simulink model "frt_dqpll"  (R2025b)
settings: Solver=ode23tb  StartTime=0.0  StopTime=simlength  FixedStep=tc  MaxStep=tc
values from neighbouring files (symbols this model uses):
  Adrso = eye(2) + Arso*ts_afe    [init_model.m]
  afe_pwm_phase_shift_mod1 = 0    [init_model.m]
  Crso = [1 0]    [init_model.m]
  delta_fht1 = 0.05    [init_model.m]
  frt_data = frt_settings(test_index, test_subindex, asymmetric_error_type, enable_frt_1, enable_frt_2, start_time_LVRT)    [init_model.m]
  grid_emu_data = grid_emulator(nominal_power, application_voltage, vp_xi_pu, vn_xi_pu, vn_eta_pu)    [init_model.m]
  i_grid_neg_eta_lim = 0.5    [init_model.m]
  i_grid_neg_eta_red_lim = 0.1    [init_model.m]
  i_grid_neg_xi_lim = 0.5    [init_model.m]
  i_grid_neg_xi_red_lim = 0.1    [init_model.m]
  i_grid_pos_eta_lim = 1    [init_model.m]
  i_grid_pos_eta_red_lim = 0.1    [init_model.m]
  ieta_neg_ref_lim = 0.5    [init_model.m]
  ieta_pos_ref_lim = 1.0    (= 1)    [init_model.m]
  ki_rc_neg_grid = ki_rc_grid    (= 35)    [init_model.m]
  ki_rc_pos_grid = ki_rc_grid    (= 35)    [init_model.m]
  kp_rc_neg_grid = kp_rc_grid    (= 0.35)    [init_model.m]
  kp_rc_pos_grid = kp_rc_grid    (= 0.35)    [init_model.m]
  Ld_fht1 = acker(Ad_fht1',Cfht1', polesd_fht1)    [init_model.m]
  Ldrso = acker(Adrso',Crso',polesdrso)'    [init_model.m]
  mavarage_filter_frequency_base_order = 2    [init_model.m]
  n1 = 2*pi*rms_perios/grid_emu_data.w_grid/ts_afe    [init_model.m]
  n10 = 2*pi*rms_perios/grid_emu_data.w_grid/ts_afe    [init_model.m]
  omega_f = grid_emu_data.w_grid    [init_model.m]
  omega_fht1 = grid_emu_data.w_grid    [init_model.m]
  pll_i1 = 80    [init_model.m]
  pll_i1_ddsrt = pll_i1    (= 80)    [init_model.m]
  pll_i1_fht = pll_i1    (= 80)    [init_model.m]
  pll_p = 1    [init_model.m]
  pll_p_ddsrt = pll_p    (= 1)    [init_model.m]
  pll_p_fht = pll_p    (= 1)    [init_model.m]
  pll_p_frt = 0.2    [init_model.m]
  start_time_LVRT = 0.75    [init_model.m]
  tc = ts_afe/400    (= 3.125e-07)    [init_model.m]
  time_gain_afe_module_1 = 1.0    (= 1)    [init_model.m]
  time_gain_inv_module_2 = 1.0    (= 1)    [init_model.m]
  ts_afe = 1/fPWM_AFE/2    (= 0.000125)    [init_model.m]
  vn_eta_pu = 0    [init_model.m]
  vn_xi_pu = 0    [init_model.m]
  vp_xi_pu = 1    [init_model.m]
  w_grid = grid_emu_data.w_grid    [init_model.m]
undefined symbols (not defined in the file or in its folder): g0_161Hz, g1_161Hz, LVRT_flt_ss_c, magnitude
libraries: fl_lib x42, nesl_utility x28, moving_average_filter x10, moving_average_filter_cc x8, cstblocks x7, discrete_time_low_pass_filter x4, simulink x3, single_phase_transformer_lib x3, linear_double_integrator_observer_ccaller x2, threephase_inductor_lib x1, power_meter_iec x1, three_phase_pwm_modulator x1
(part 4 of 6)

== system frt_dqpll/AFE_control/afe_control/grid_voltage_phase_lock_loops/dq_pll_ccaller/first_harmonic_tracker_phase_u ==
  u : Inport
  Bus Selector : BusSelector  OutputSignals=output_pu_hat
  C Caller : CCaller  FunctionName=first_harmonic_tracker_process_simulink  PortSpecificationStruct="%)30     .    B \\   8    (     @         %    \"     D    !     0         %  0 \"0    $    _    07)G3F%M90  4&]R=$YA;64 4V-O<&4     26YD97@     5'EP90      4VEZ90      27-';&]B86P   X    P    !@    @    $          4    (     0    ,    !         !   P!O=70 #@   #     &    \"     0         !0    @    !     P    $         $  # &]U=  .    .     8    (    !          %    \"     $    &     0         0  ...(+4988 chars)"
  Constant : Constant  Value=ts_afe
  Constant1 : Constant  Value=0
  Constant4 : Constant  Value=omega_fht1
  Constant5 : Constant  Value=delta_fht1
  Constant6 : Constant  Value=Ld_fht1(1)
  Constant7 : Constant  Value=Ld_fht1(2)
  Data Type Conversion{1..2,6..9} (6 alike) : DataTypeConversion  OutDataTypeStr=single  SaturateOnIntegerOverflow=off  RndMeth=Floor
  Data Type Conversion3 : DataTypeConversion  OutDataTypeStr=uint8  SaturateOnIntegerOverflow=off  RndMeth=Floor
  Data Type Conversion4 : DataTypeConversion  OutDataTypeStr=double  SaturateOnIntegerOverflow=off  RndMeth=Floor
  Data Type Conversion5 : DataTypeConversion  OutDataTypeStr=uint8  SaturateOnIntegerOverflow=off  RndMeth=Floor
  Step : Step  Time=0.0125  Before=1  After=0
  u_hat : Outport
  wires:
  Data Type Conversion4/1 -> u_hat/1
  Data Type Conversion3/1 -> C Caller/1
  Data Type Conversion1/1 -> C Caller/3
  Data Type Conversion2/1 -> C Caller/2
  C Caller/1 -> Bus Selector/1
  Bus Selector/1 -> Data Type Conversion4/1  "<output_pu_hat>"
  Step/1 -> Data Type Conversion3/1
  u/1 -> Data Type Conversion2/1
  Constant/1 -> Data Type Conversion1/1
  Constant1/1 -> Data Type Conversion5/1
  Constant4/1 -> Data Type Conversion6/1
  Constant6/1 -> Data Type Conversion8/1
  Constant7/1 -> Data Type Conversion9/1
  Constant5/1 -> Data Type Conversion7/1
  Data Type Conversion5/1 -> C Caller/8
  Data Type Conversion6/1 -> C Caller/4
  Data Type Conversion7/1 -> C Caller/5
  Data Type Conversion8/1 -> C Caller/6
  Data Type Conversion9/1 -> C Caller/7

== system frt_dqpll/AFE_control/afe_control/grid_voltage_phase_lock_loops/dq_pll_ccaller/first_harmonic_tracker_phase_v ==
  u : Inport
  Bus Selector : BusSelector  OutputSignals=output_pu_hat
  C Caller : CCaller  FunctionName=first_harmonic_tracker_process_simulink  PortSpecificationStruct="%)30     .    B \\   8    (     @         %    \"     D    !     0         %  0 \"0    $    _    07)G3F%M90  4&]R=$YA;64 4V-O<&4     26YD97@     5'EP90      4VEZ90      27-';&]B86P   X    P    !@    @    $          4    (     0    ,    !         !   P!O=70 #@   #     &    \"     0         !0    @    !     P    $         $  # &]U=  .    .     8    (    !          %    \"     $    &     0         0  ...(+4988 chars)"
  Constant : Constant  Value=ts_afe
  Constant1 : Constant  Value=2
  Constant4 : Constant  Value=omega_fht1
  Constant5 : Constant  Value=delta_fht1
  Constant6 : Constant  Value=Ld_fht1(1)
  Constant7 : Constant  Value=Ld_fht1(2)
  Data Type Conversion{1..2,6..9} (6 alike) : DataTypeConversion  OutDataTypeStr=single  SaturateOnIntegerOverflow=off  RndMeth=Floor
  Data Type Conversion3 : DataTypeConversion  OutDataTypeStr=uint8  SaturateOnIntegerOverflow=off  RndMeth=Floor
  Data Type Conversion4 : DataTypeConversion  OutDataTypeStr=double  SaturateOnIntegerOverflow=off  RndMeth=Floor
  Data Type Conversion5 : DataTypeConversion  OutDataTypeStr=uint8  SaturateOnIntegerOverflow=off  RndMeth=Floor
  Step : Step  Time=0.0125  Before=1  After=0
  u_hat : Outport
  wires:
  Data Type Conversion9/1 -> C Caller/7
  Data Type Conversion8/1 -> C Caller/6
  Data Type Conversion7/1 -> C Caller/5
  Data Type Conversion6/1 -> C Caller/4
  Data Type Conversion5/1 -> C Caller/8
  Constant5/1 -> Data Type Conversion7/1
  Constant7/1 -> Data Type Conversion9/1
  Constant6/1 -> Data Type Conversion8/1
  Constant4/1 -> Data Type Conversion6/1
  Constant1/1 -> Data Type Conversion5/1
  Constant/1 -> Data Type Conversion1/1
  u/1 -> Data Type Conversion2/1
  Step/1 -> Data Type Conversion3/1
  Bus Selector/1 -> Data Type Conversion4/1  "<output_pu_hat>"
  C Caller/1 -> Bus Selector/1
  Data Type Conversion2/1 -> C Caller/2
  Data Type Conversion1/1 -> C Caller/3
  Data Type Conversion3/1 -> C Caller/1
  Data Type Conversion4/1 -> u_hat/1

== system frt_dqpll/AFE_control/afe_control/grid_voltage_phase_lock_loops/dq_pll_ccaller/first_harmonic_tracker_phase_w ==
  u : Inport
  Bus Selector : BusSelector  OutputSignals=output_pu_hat
  C Caller : CCaller  FunctionName=first_harmonic_tracker_process_simulink  PortSpecificationStruct="%)30     .    B \\   8    (     @         %    \"     D    !     0         %  0 \"0    $    _    07)G3F%M90  4&]R=$YA;64 4V-O<&4     26YD97@     5'EP90      4VEZ90      27-';&]B86P   X    P    !@    @    $          4    (     0    ,    !         !   P!O=70 #@   #     &    \"     0         !0    @    !     P    $         $  # &]U=  .    .     8    (    !          %    \"     $    &     0         0  ...(+4988 chars)"
  Constant : Constant  Value=ts_afe
  Constant1 : Constant  Value=4
  Constant4 : Constant  Value=omega_fht1
  Constant5 : Constant  Value=delta_fht1
  Constant6 : Constant  Value=Ld_fht1(1)
  Constant7 : Constant  Value=Ld_fht1(2)
  Data Type Conversion{1..2,6..9} (6 alike) : DataTypeConversion  OutDataTypeStr=single  SaturateOnIntegerOverflow=off  RndMeth=Floor
  Data Type Conversion3 : DataTypeConversion  OutDataTypeStr=uint8  SaturateOnIntegerOverflow=off  RndMeth=Floor
  Data Type Conversion4 : DataTypeConversion  OutDataTypeStr=double  SaturateOnIntegerOverflow=off  RndMeth=Floor
  Data Type Conversion5 : DataTypeConversion  OutDataTypeStr=uint8  SaturateOnIntegerOverflow=off  RndMeth=Floor
  Step : Step  Time=0.0125  Before=1  After=0
  u_hat : Outport
  wires:
  Data Type Conversion4/1 -> u_hat/1
  Data Type Conversion3/1 -> C Caller/1
  Data Type Conversion1/1 -> C Caller/3
  Data Type Conversion2/1 -> C Caller/2
  C Caller/1 -> Bus Selector/1
  Bus Selector/1 -> Data Type Conversion4/1  "<output_pu_hat>"
  Step/1 -> Data Type Conversion3/1
  u/1 -> Data Type Conversion2/1
  Constant/1 -> Data Type Conversion1/1
  Constant1/1 -> Data Type Conversion5/1
  Constant4/1 -> Data Type Conversion6/1
  Constant6/1 -> Data Type Conversion8/1
  Constant7/1 -> Data Type Conversion9/1
  Constant5/1 -> Data Type Conversion7/1
  Data Type Conversion5/1 -> C Caller/8
  Data Type Conversion6/1 -> C Caller/4
  Data Type Conversion7/1 -> C Caller/5
  Data Type Conversion8/1 -> C Caller/6
  Data Type Conversion9/1 -> C Caller/7

== system frt_dqpll/AFE_control/afe_control/grid_voltage_sequences/voltage_sequence_avg/average_filter ==
  v_grid_pos_xi : Inport
  v_grid_pos_eta : Inport  Port=2
  v_grid_neg_xi : Inport  Port=3
  v_grid_neg_eta : Inport  Port=4
  Abs : Abs  SaturateOnIntegerOverflow=off
  Gain : Gain  Gain=grid_emu_data.omega_grid_nom*mavarage_filter_frequency_base_order
  Saturation : Saturate  UpperLimit=2  LowerLimit=0.1
  dmavg_flt{,1..3} (4 alike) : moving_average_filter/dmavg_flt  ts=ts_afe  enable_time=dmavg_filter_enable_time
  v_grid_pos_xi_avg : Outport
  v_grid_pos_eta_avg : Outport  Port=2
  v_grid_neg_xi_avg : Outport  Port=3
  v_grid_neg_eta_avg : Outport  Port=4
  wires:
  v_grid_neg_eta/1 -> dmavg_flt3/1
  v_grid_neg_xi/1 -> dmavg_flt2/1
  v_grid_pos_eta/1 -> dmavg_flt1/1
  dmavg_flt3/1 -> v_grid_neg_eta_avg/1
  dmavg_flt2/1 -> v_grid_neg_xi_avg/1
  dmavg_flt1/1 -> v_grid_pos_eta_avg/1
  Gain/1 -> dmavg_flt/2, dmavg_flt1/2, dmavg_flt2/2, dmavg_flt3/2
  dmavg_flt/1 -> v_grid_pos_xi_avg/1
  v_grid_pos_xi/1 -> dmavg_flt/1
  Abs/1 -> Saturation/1
  [omega_grid_pll_pu_mod1] -> Abs/1
  Saturation/1 -> Gain/1

== system frt_dqpll/AFE_control/afe_control/grid_voltage_sequences/voltage_sequence_avg/average_filter_ccaller ==
  v_grid_pos_xi : Inport
  v_grid_pos_eta : Inport  Port=2
  v_grid_neg_xi : Inport  Port=3
  v_grid_neg_eta : Inport  Port=4
  Abs : Abs  SaturateOnIntegerOverflow=off
  Gain : Gain  Gain=grid_emu_data.omega_grid_nom*mavarage_filter_frequency_base_order
  Saturation : Saturate  UpperLimit=2  LowerLimit=0.1
  dmavg_flt : moving_average_filter_cc/dmavg_flt  instance=0  ts=ts_afe  enable_time=dmavg_filter_enable_time
  dmavg_flt1 : moving_average_filter_cc/dmavg_flt  instance=1  ts=ts_afe  enable_time=dmavg_filter_enable_time
  dmavg_flt2 : moving_average_filter_cc/dmavg_flt  instance=2  ts=ts_afe  enable_time=dmavg_filter_enable_time
  dmavg_flt3 : moving_average_filter_cc/dmavg_flt  instance=3  ts=ts_afe  enable_time=dmavg_filter_enable_time
  v_grid_pos_xi_avg : Outport
  v_grid_pos_eta_avg : Outport  Port=2
  v_grid_neg_xi_avg : Outport  Port=3
  v_grid_neg_eta_avg : Outport  Port=4
  wires:
  v_grid_pos_xi/1 -> dmavg_flt/1
  dmavg_flt/1 -> v_grid_pos_xi_avg/1
  dmavg_flt1/1 -> v_grid_pos_eta_avg/1
  dmavg_flt2/1 -> v_grid_neg_xi_avg/1
  dmavg_flt3/1 -> v_grid_neg_eta_avg/1
  v_grid_pos_eta/1 -> dmavg_flt1/1
  v_grid_neg_xi/1 -> dmavg_flt2/1
  v_grid_neg_eta/1 -> dmavg_flt3/1
  Abs/1 -> Saturation/1
  Saturation/1 -> Gain/1
  [omega_grid_pll_pu_mod1] -> Abs/1
  Gain/1 -> dmavg_flt/2, dmavg_flt1/2, dmavg_flt3/2, dmavg_flt2/2

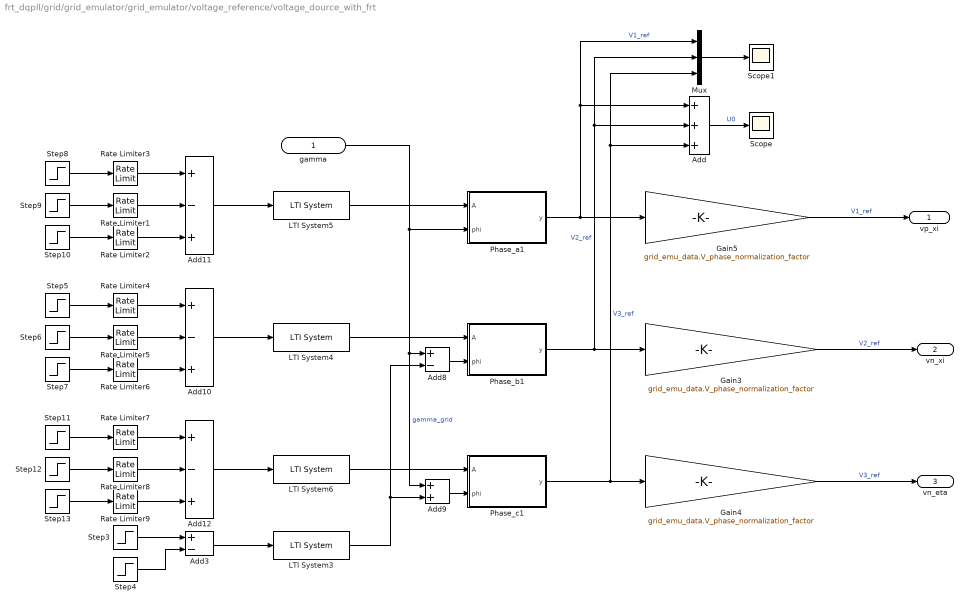
== system frt_dqpll/grid/grid_emulator/grid_emulator/voltage_reference/voltage_dource_with_frt ==
  gamma : Inport
  Add : Sum  Inputs=+++
  Add10 : Sum  Inputs=+-+
  Add11 : Sum  Inputs=+-+
  Add12 : Sum  Inputs=+-+
  Add3 : Sum  Inputs=+-
  Add8 : Sum  Inputs=+-
  Add9 : Sum
  Gain3 : Gain  Gain=grid_emu_data.V_phase_normalization_factor
  Gain4 : Gain  Gain=grid_emu_data.V_phase_normalization_factor
  Gain5 : Gain  Gain=grid_emu_data.V_phase_normalization_factor
  LTI System{3..6} (4 alike) : cstblocks/LTI System  sys=LVRT_flt_ss_c  IC=[0]  PadeOrder=0
  Mux : Mux  Inputs=3
  Phase_a1 : MATLAB Function  TreatAsAtomicUnit=on
  Phase_b1 : MATLAB Function  TreatAsAtomicUnit=on
  Phase_c1 : MATLAB Function  TreatAsAtomicUnit=on
  Rate Limiter{1..9} (9 alike) : RateLimiter  RisingSlewLimit=grid_emu_data.Vemu_ref_norm/frt_data.t_ramp  FallingSlewLimit=-grid_emu_data.Vemu_ref_norm/frt_data.t_ramp  SampleTimeMode=inherited
  Scope : Scope
      settings: ActiveDisplayYMinimum=-1E-15  ActiveDisplayYMaximum=8E-16
  Scope1 : Scope
      settings: ActiveDisplayYMinimum=-1.25511  ActiveDisplayYMaximum=1.25511
  Step10 : Step  Time=frt_data.end_time_LVRT  After=grid_emu_data.Vemu_ref_norm*(1-frt_data.Amplitude_U)  SampleTime=0
  Step11 : Step  Time=0  After=grid_emu_data.Vemu_ref_norm  SampleTime=0
  Step12 : Step  Time=frt_data.start_time_LVRT  After=grid_emu_data.Vemu_ref_norm*(1-frt_data.Amplitude_W)  SampleTime=0
  Step13 : Step  Time=frt_data.end_time_LVRT  After=grid_emu_data.Vemu_ref_norm*(1-frt_data.Amplitude_W)  SampleTime=0
  Step3 : Step  Time=frt_data.start_time_LVRT  After=frt_data.Phase_shift  SampleTime=0
  Step4 : Step  Time=frt_data.end_time_LVRT  After=frt_data.Phase_shift  SampleTime=0
  Step5 : Step  Time=0  After=grid_emu_data.Vemu_ref_norm  SampleTime=0
  Step6 : Step  Time=frt_data.start_time_LVRT  After=grid_emu_data.Vemu_ref_norm*(1-frt_data.Amplitude_V)  SampleTime=0
  Step7 : Step  Time=frt_data.end_time_LVRT  After=grid_emu_data.Vemu_ref_norm*(1-frt_data.Amplitude_V)  SampleTime=0
  Step8 : Step  Time=0  After=grid_emu_data.Vemu_ref_norm  SampleTime=0
  Step9 : Step  Time=frt_data.start_time_LVRT  After=grid_emu_data.Vemu_ref_norm*(1-frt_data.Amplitude_U)  SampleTime=0
  vp_xi : Outport  VectorParamsAs1DForOutWhenUnconnected=off
  vn_xi : Outport  Port=2  VectorParamsAs1DForOutWhenUnconnected=off
  vn_eta : Outport  Port=3  VectorParamsAs1DForOutWhenUnconnected=off
  wires:
  Phase_c1/1(y) -> Mux/3, Add/3, Gain4/1  "V3_ref"
  LTI System6/1 -> Phase_c1/1(A)
  gamma/1 -> Add9/1, Add8/1, Phase_a1/2(phi)  "gamma_grid"
  Add9/1 -> Phase_c1/2(phi)
  Add8/1 -> Phase_b1/2(phi)
  Phase_b1/1(y) -> Mux/2, Add/2, Gain3/1  "V2_ref"
  Phase_a1/1(y) -> Mux/1, Add/1, Gain5/1  "V1_ref"
  LTI System4/1 -> Phase_b1/1(A)
  Step5/1 -> Rate Limiter4/1
  Step6/1 -> Rate Limiter5/1
  Step7/1 -> Rate Limiter6/1
  Add10/1 -> LTI System4/1
  Step8/1 -> Rate Limiter3/1
  Add11/1 -> LTI System5/1
  Step9/1 -> Rate Limiter1/1
  Step10/1 -> Rate Limiter2/1
  LTI System5/1 -> Phase_a1/1(A)
  Add12/1 -> LTI System6/1
  Rate Limiter3/1 -> Add11/1
  Rate Limiter1/1 -> Add11/2
  Rate Limiter2/1 -> Add11/3
  Rate Limiter4/1 -> Add10/1
  Rate Limiter5/1 -> Add10/2
  Rate Limiter6/1 -> Add10/3
  Step12/1 -> Rate Limiter8/1
  Rate Limiter8/1 -> Add12/2
  Step13/1 -> Rate Limiter9/1
  Rate Limiter9/1 -> Add12/3
  Step11/1 -> Rate Limiter7/1
  Rate Limiter7/1 -> Add12/1
  Gain5/1 -> vp_xi/1  "V1_ref"
  Gain3/1 -> vn_xi/1  "V2_ref"
  Gain4/1 -> vn_eta/1  "V3_ref"
  Add3/1 -> LTI System3/1
  Step3/1 -> Add3/1
  Step4/1 -> Add3/2
  LTI System3/1 -> Add9/2, Add8/2
  Add/1 -> Scope/1  "U0"
  Mux/1 -> Scope1/1

== system frt_dqpll/grid/grid_emulator/three_phase_voltage_source_with_frt_emulator/three_phase_voltage_source_emulator/phase_gen1 ==
  Constant4 : Constant  Value=nominal_frequency_m*2*pi
  Integrator : Integrator
  bounder : MATLAB Function  TreatAsAtomicUnit=on  SystemSampleTime=ts_afe
  grid_emu_phase : Outport  VectorParamsAs1DForOutWhenUnconnected=off
  tag scope: gamma_grid_emulator=scoped, omega_grid_emulator=scoped
  wires:
  Integrator/1 -> bounder/1(u)
  Constant4/1 -> Integrator/1, [omega_grid_emulator]
  bounder/1(y) -> grid_emu_phase/1, [gamma_grid_emulator]  "grid_emu_phase"

== system frt_dqpll/grid/grid_emulator/three_phase_voltage_source_with_frt_emulator/three_phase_voltage_source_emulator/voltage_reference1 ==
  grid_emu_phase : Inport
  Vxi_p : Inport  Port=2
  Vxi_n : Inport  Port=3
  Veta_n : Inport  Port=4
  Constant2 : Constant  Value=0
  Sum1 : Sum  Inputs=|++
  Sum4 : Sum  Inputs=|++
  Variant Source : VariantSource  VariantControls={enable_frt_2_m == 1, enable_frt_1_m == 1}
  Variant Source1 : VariantSource  VariantControls={enable_frt_2_m == 1, enable_frt_1_m == 1}
  Variant Source2 : VariantSource  VariantControls={enable_frt_2_m == 1, enable_frt_1_m == 1}
  alphabeta2abc : MATLAB Function  TreatAsAtomicUnit=on  SystemSampleTime=ts_afe
  voltage_dource_with_frt : Subsystem
  xieta2alphabeta_neg : MATLAB Function  TreatAsAtomicUnit=on  SystemSampleTime=ts_afe
  xieta2alphabeta_pos : MATLAB Function  TreatAsAtomicUnit=on  SystemSampleTime=ts_afe
  V1_ref : Outport  VectorParamsAs1DForOutWhenUnconnected=off
  V2_ref : Outport  Port=2  VectorParamsAs1DForOutWhenUnconnected=off
  V3_ref : Outport  Port=3  VectorParamsAs1DForOutWhenUnconnected=off
  wires:
  [V3_ref_xieta] -> Variant Source2/1
  [V3_ref_abc] -> Variant Source2/2
  Variant Source2/1 -> V3_ref/1
  [V2_ref_abc] -> Variant Source1/2
  [V2_ref_xieta] -> Variant Source1/1
  Variant Source1/1 -> V2_ref/1
  [V1_ref_abc] -> Variant Source/2
  [V1_ref_xieta] -> Variant Source/1
  voltage_dource_with_frt/1(vp_xi) -> [V1_ref_abc]
  voltage_dource_with_frt/2(vn_xi) -> [V2_ref_abc]
  voltage_dource_with_frt/3(vn_eta) -> [V3_ref_abc]
  alphabeta2abc/3(c) -> [V3_ref_xieta]
  alphabeta2abc/2(b) -> [V2_ref_xieta]
  alphabeta2abc/1(a) -> [V1_ref_xieta]
  Variant Source/1 -> V1_ref/1
  Veta_n/1 -> xieta2alphabeta_neg/2(eta)
  Vxi_n/1 -> xieta2alphabeta_neg/1(xi)
  Constant2/1 -> xieta2alphabeta_pos/2(eta)
  Vxi_p/1 -> xieta2alphabeta_pos/1(xi)
  grid_emu_phase/1 -> xieta2alphabeta_pos/3(gamma), xieta2alphabeta_neg/3(gamma), voltage_dource_with_frt/1(gamma)
  xieta2alphabeta_neg/2(beta) -> Sum4/2
  xieta2alphabeta_neg/1(alpha) -> Sum1/2
  Sum4/1 -> alphabeta2abc/2(beta)
  xieta2alphabeta_pos/2(beta) -> Sum4/1
  Sum1/1 -> alphabeta2abc/1(alpha)
  xieta2alphabeta_pos/1(alpha) -> Sum1/1

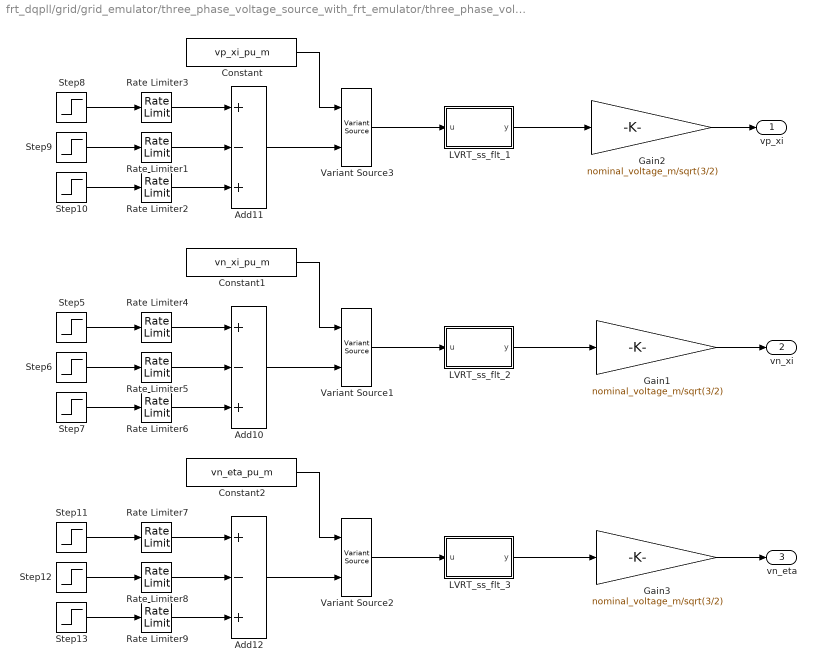
== system frt_dqpll/grid/grid_emulator/three_phase_voltage_source_with_frt_emulator/three_phase_voltage_source_emulator/voltage_source ==
  Add10 : Sum  Inputs=+-+
  Add11 : Sum  Inputs=+-+
  Add12 : Sum  Inputs=+-+
  Constant : Constant  Value=vp_xi_pu_m
  Constant1 : Constant  Value=vn_xi_pu_m
  Constant2 : Constant  Value=vn_eta_pu_m
  Gain1 : Gain  Gain=nominal_voltage_m/sqrt(3/2)
  Gain2 : Gain  Gain=nominal_voltage_m/sqrt(3/2)
  Gain3 : Gain  Gain=nominal_voltage_m/sqrt(3/2)
  LVRT_ss_flt_1 : Subsystem
  LVRT_ss_flt_2 : Subsystem
  LVRT_ss_flt_3 : Subsystem
  Rate Limiter{1..9} (9 alike) : RateLimiter  RisingSlewLimit=Vemu_ref_norm_m/t_ramp_m  FallingSlewLimit=-Vemu_ref_norm_m/t_ramp_m  SampleTimeMode=inherited
  Step10 : Step  Time=end_time_LVRT_m  After=vp_xi_pu_m*deepPOSxi_m  SampleTime=0
  Step11 : Step  Time=0  After=vn_eta_pu_m  SampleTime=0
  Step12 : Step  Time=start_time_LVRT_m  After=deepNEGeta_m  SampleTime=0
  Step13 : Step  Time=end_time_LVRT_m  After=deepNEGeta_m  SampleTime=0
  Step5 : Step  Time=0  After=vn_xi_pu_m  SampleTime=0
  Step6 : Step  Time=start_time_LVRT_m  After=deepNEGxi_m  SampleTime=0
  Step7 : Step  Time=end_time_LVRT_m  After=deepNEGxi_m  SampleTime=0
  Step8 : Step  Time=0  After=vp_xi_pu_m  SampleTime=0
  Step9 : Step  Time=start_time_LVRT_m  After=vp_xi_pu_m*deepPOSxi_m  SampleTime=0
  Variant Source1 : VariantSource  VariantControls={(enable_frt_1_m || enable_frt_2_m) == 0, (enable_frt_1_m || enable_frt_2_m) == 1}
  Variant Source2 : VariantSource  VariantControls={(enable_frt_1_m || enable_frt_2_m) == 0, (enable_frt_1_m || enable_frt_2_m) == 1}
  Variant Source3 : VariantSource  VariantControls={(enable_frt_1_m || enable_frt_2_m) == 0, (enable_frt_1_m || enable_frt_2_m) == 1}
  vp_xi : Outport  VectorParamsAs1DForOutWhenUnconnected=off
  vn_xi : Outport  Port=2  VectorParamsAs1DForOutWhenUnconnected=off
  vn_eta : Outport  Port=3  VectorParamsAs1DForOutWhenUnconnected=off
  wires:
  LVRT_ss_flt_3/1(y) -> Gain3/1
  LVRT_ss_flt_2/1(y) -> Gain1/1
  Variant Source2/1 -> LVRT_ss_flt_3/1(u)
  Variant Source1/1 -> LVRT_ss_flt_2/1(u)
  LVRT_ss_flt_1/1(y) -> Gain2/1
  Constant2/1 -> Variant Source2/1
  Add12/1 -> Variant Source2/2
  Constant1/1 -> Variant Source1/1
  Add10/1 -> Variant Source1/2
  Constant/1 -> Variant Source3/1
  Variant Source3/1 -> LVRT_ss_flt_1/1(u)
  Add11/1 -> Variant Source3/2
  Step13/1 -> Rate Limiter9/1
  Step10/1 -> Rate Limiter2/1
  Rate Limiter6/1 -> Add10/3
  Rate Limiter4/1 -> Add10/1
  Rate Limiter9/1 -> Add12/3
  Rate Limiter8/1 -> Add12/2
  Rate Limiter3/1 -> Add11/1
  Step9/1 -> Rate Limiter1/1
  Rate Limiter1/1 -> Add11/2
  Step11/1 -> Rate Limiter7/1
  Step12/1 -> Rate Limiter8/1
  Step8/1 -> Rate Limiter3/1
  Rate Limiter7/1 -> Add12/1
  Step5/1 -> Rate Limiter4/1
  Rate Limiter5/1 -> Add10/2
  Step6/1 -> Rate Limiter5/1
  Step7/1 -> Rate Limiter6/1
  Rate Limiter2/1 -> Add11/3
  Gain3/1 -> vn_eta/1
  Gain1/1 -> vn_xi/1
  Gain2/1 -> vp_xi/1

== system frt_dqpll/AFE_control/afe_control/grid_voltage_phase_lock_loops/DDSRF-PLL/pll_stageA/filter_and_transformation ==
  ug_a : Inport
  ug_b : Inport  Port=2
  ug_c : Inport  Port=3
  abc2alphabeta : MATLAB Function  TreatAsAtomicUnit=on
  first_harmonic_tracker : Scope  NumInputPorts=3
      settings: ActiveDisplayYMinimum=-1.7184470891952515  ActiveDisplayYMaximum=1.8384636640548706  DataLoggingVariableName=ScopeData3
  first_harmonic_tracker_phase_u : Subsystem
  first_harmonic_tracker_phase_v : Subsystem
  first_harmonic_tracker_phase_w : Subsystem
  ug_alpha : Outport  VectorParamsAs1DForOutWhenUnconnected=off
  ug_beta : Outport  Port=2  VectorParamsAs1DForOutWhenUnconnected=off
  wires:
  abc2alphabeta/1(alpha) -> ug_alpha/1  "u_grid_alpha"
  abc2alphabeta/2(beta) -> ug_beta/1  "u_grid_beta"
  first_harmonic_tracker_phase_u/1(u_hat) -> first_harmonic_tracker/1, abc2alphabeta/1(a)  "tracker_phase_u"
  first_harmonic_tracker_phase_w/1(u_hat) -> first_harmonic_tracker/3, abc2alphabeta/3(c)  "tracker_phase_w"
  first_harmonic_tracker_phase_v/1(u_hat) -> first_harmonic_tracker/2, abc2alphabeta/2(b)  "tracker_phase_v"
  ug_a/1 -> first_harmonic_tracker_phase_u/1(u)
  ug_b/1 -> first_harmonic_tracker_phase_v/1(u)
  ug_c/1 -> first_harmonic_tracker_phase_w/1(u)

== system frt_dqpll/AFE_control/afe_control/grid_voltage_phase_lock_loops/DDSRF-PLL/pll_stageA/sequences ==
  u_grid_alpha : Inport
  u_grid_beta : Inport  Port=2
  phase_angle : Inport  Port=3
  ddsrf : Subsystem
  u_grid_pos_xi : Outport
  u_grid_pos_eta : Outport  Port=2
  wires:
  phase_angle/1 -> ddsrf/3(phase_angle)  "phase_angle"
  u_grid_beta/1 -> ddsrf/2(u_grid_beta)  "u_grid_beta"
  u_grid_alpha/1 -> ddsrf/1(u_grid_alpha)  "u_grid_alpha"
  ddsrf/4(u_grid_neg_eta) -> u_grid_pos_eta/1  "u_grid_pos_eta"
  ddsrf/3(u_grid_neg_xi) -> u_grid_pos_xi/1  "u_grid_pos_xi"

== system frt_dqpll/AFE_control/afe_control/grid_voltage_phase_lock_loops/DDSRF-PLL/pll_stageB/double_integrator_observer ==
  theta : Inport
  Gain : Gain  Gain=Ldrso  Multiplication=Matrix(K*u)
  Gain1 : Gain  Gain=Adrso  Multiplication=Matrix(K*u)
  Gain2 : Gain  Gain=Crso  Multiplication=Matrix(K*u)
  Selector : Selector  InputPortWidth=2  IndexOptions=Index vector (dialog)  Indices=2  OutputSizes=1
  Sum : Sum  Inputs=-+|
  Sum1 : Sum  Inputs=|++
  Unit Delay : UnitDelay  SampleTime=-1  HasFrameUpgradeWarning=on
  bounder1 : MATLAB Function  TreatAsAtomicUnit=on
  bounder2 : MATLAB Function  TreatAsAtomicUnit=on
  omega_hat : Outport
  wires:
  bounder2/1(y) -> Sum/1  "theta_hat_bounded"
  bounder1/1(y) -> Gain/1  "e_bounded"
  theta/1 -> Sum/2  "theta"
  Unit Delay/1 -> Gain2/1, Selector/1, Gain1/1
  Sum/1 -> bounder1/1(u)  "e"
  Sum1/1 -> Unit Delay/1
  Gain1/1 -> Sum1/2
  Gain2/1 -> bounder2/1(u)  "theta_hat"
  Selector/1 -> omega_hat/1
  Gain/1 -> Sum1/1

== system frt_dqpll/AFE_control/afe_control/grid_voltage_phase_lock_loops/FHT-PLL/pll_stageA/filter_and_transformation ==
  ug_a : Inport
  ug_b : Inport  Port=2
  ug_c : Inport  Port=3
  Bus Creator : BusCreator  Inputs=2
  Bus Creator1 : BusCreator  Inputs=3
  Bus Creator2 : BusCreator  Inputs=2
  Bus Creator3 : BusCreator  Inputs=3
  Bus Creator4 : BusCreator  Inputs=3
  FHTalpha : Subsystem
  FHTbeta : Subsystem
  FHTdqPLL : Scope  NumInputPorts=2
      settings: ActiveDisplayYMinimum=-1.5258214459194912  ActiveDisplayYMaximum=1.5258228058860459  DataLoggingVariableName=ScopeData12
  Gain : Gain  Gain=-1/2
  Gain1 : Gain  Gain=-1/2
  Sum : Sum  Inputs=|++
  Sum1 : Sum  Inputs=-+|
  To Workspace1 : ToWorkspace  VariableName=ugd_alpha_sim  SampleTime=-1
      settings: MaxDataPoints=Ns_afe
  To Workspace2 : ToWorkspace  VariableName=ugd_beta_sim  SampleTime=-1
      settings: MaxDataPoints=Ns_afe
  To Workspace3 : ToWorkspace  VariableName=u_fht_alpha_sim  SampleTime=-1
      settings: MaxDataPoints=Ns_afe
  To Workspace4 : ToWorkspace  VariableName=v_fht_alpha_sim  SampleTime=-1
      settings: MaxDataPoints=Ns_afe
  To Workspace5 : ToWorkspace  VariableName=u_fhtsr_alpha_sim  SampleTime=-1
      settings: MaxDataPoints=Ns_afe
  To Workspace6 : ToWorkspace  VariableName=u_fhtsr_beta_sim  SampleTime=-1
      settings: MaxDataPoints=Ns_afe
  To Workspace7 : ToWorkspace  VariableName=u_fht_beta_sim  SampleTime=-1
      settings: MaxDataPoints=Ns_afe
  To Workspace8 : ToWorkspace  VariableName=v_fht_beta_sim  SampleTime=-1
      settings: MaxDataPoints=Ns_afe
  To Workspace9 : ToWorkspace  VariableName=ugd_abc_grid_sim  SampleTime=-1
      settings: MaxDataPoints=Ns_afe
  abc2alphabeta : MATLAB Function  TreatAsAtomicUnit=on
  grid_voltages : Scope  NumInputPorts=3
      settings: ActiveDisplayYMinimum=-1.3618303835391998  ActiveDisplayYMaximum=1.3331545889377594  DataLoggingVariableName=ScopeData13
  ug_alpha : Outport  VectorParamsAs1DForOutWhenUnconnected=off
  ug_beta : Outport  Port=2  VectorParamsAs1DForOutWhenUnconnected=off
  wires:
  ug_b/1 -> Bus Creator3/2, grid_voltages/2, abc2alphabeta/2(b)  "ugd_b"
  ug_c/1 -> Bus Creator3/3, grid_voltages/3, abc2alphabeta/3(c)  "ugd_c"
  ug_a/1 -> Bus Creator3/1, grid_voltages/1, abc2alphabeta/1(a)  "ugd_a"
  abc2alphabeta/1(alpha) -> To Workspace1/1, FHTalpha/1(u), Bus Creator4/1  "u_grid_alpha"
  abc2alphabeta/2(beta) -> FHTbeta/1(u), To Workspace2/1, Bus Creator1/1  "u_grid_beta"
  FHTalpha/1(ud_hat) -> To Workspace3/1, Bus Creator/1, Sum/1  "u_fht_alpha"
  Sum/1 -> Gain/1
  FHTbeta/1(ud_hat) -> Sum1/2, To Workspace7/1, Bus Creator2/1  "u_fht_beta"
  Sum1/1 -> Gain1/1
  Gain1/1 -> Bus Creator1/3, To Workspace6/1, ug_beta/1  "u_fhtsr_beta"
  Gain/1 -> Bus Creator4/3, To Workspace5/1, ug_alpha/1  "u_fhtsr_alpha"
  FHTbeta/2(uq_hat) -> Sum/2, To Workspace8/1, Bus Creator2/2  "v_fht_beta"
  FHTalpha/2(uq_hat) -> Sum1/1, To Workspace4/1, Bus Creator/2  "v_fht_alpha"
  Bus Creator1/1 -> FHTdqPLL/2
  Bus Creator4/1 -> FHTdqPLL/1
  Bus Creator/1 -> Bus Creator4/2  "FHTalpha"
  Bus Creator2/1 -> Bus Creator1/2  "FHTbeta"
  Bus Creator3/1 -> To Workspace9/1

== system frt_dqpll/AFE_control/afe_control/grid_voltage_phase_lock_loops/FHT-PLL/pll_stageA/sequences ==
  u_grid_alpha : Inport
  u_grid_beta : Inport  Port=2
  phase_angle : Inport  Port=3
  alphabeta2xieta : MATLAB Function  TreatAsAtomicUnit=on
  u_grid_xi : Outport
  u_grid_eta : Outport  Port=2
  wires:
  alphabeta2xieta/1(xi) -> u_grid_xi/1  "u_grid_xi"
  alphabeta2xieta/2(eta) -> u_grid_eta/1  "u_grid_eta"
  u_grid_alpha/1 -> alphabeta2xieta/1(alpha)  "u_grid_alpha"
  u_grid_beta/1 -> alphabeta2xieta/2(beta)  "u_grid_beta"
  phase_angle/1 -> alphabeta2xieta/3(gamma)  "phase_angle"

== system frt_dqpll/AFE_control/afe_control/grid_voltage_phase_lock_loops/FHT-PLL/pll_stageB/double_integrator_observer ==
  theta : Inport
  Gain : Gain  Gain=Ldrso  Multiplication=Matrix(K*u)
  Gain1 : Gain  Gain=Adrso  Multiplication=Matrix(K*u)
  Gain2 : Gain  Gain=Crso  Multiplication=Matrix(K*u)
  Selector : Selector  InputPortWidth=2  IndexOptions=Index vector (dialog)  Indices=2  OutputSizes=1
  Sum : Sum  Inputs=-+|
  Sum1 : Sum  Inputs=|++
  Unit Delay : UnitDelay  SampleTime=-1  HasFrameUpgradeWarning=on
  bounder1 : MATLAB Function  TreatAsAtomicUnit=on
  bounder2 : MATLAB Function  TreatAsAtomicUnit=on
  omega_hat : Outport
  wires:
  Gain/1 -> Sum1/1
  Selector/1 -> omega_hat/1
  Gain2/1 -> bounder2/1(u)  "theta_hat"
  Gain1/1 -> Sum1/2
  Sum1/1 -> Unit Delay/1
  Sum/1 -> bounder1/1(u)  "e"
  Unit Delay/1 -> Gain1/1, Selector/1, Gain2/1
  theta/1 -> Sum/2  "theta"
  bounder1/1(y) -> Gain/1  "e_bounded"
  bounder2/1(y) -> Sum/1  "theta_hat_bounded"

== system frt_dqpll/AFE_control/afe_control/grid_voltage_phase_lock_loops/dq_pll/pll_stageA/mormalization_and_transformation ==
  ug_a : Inport
  ug_b : Inport  Port=2
  ug_c : Inport  Port=3
  abc2alphabeta : MATLAB Function  TreatAsAtomicUnit=on
  ug_alpha : Outport  VectorParamsAs1DForOutWhenUnconnected=off
  ug_beta : Outport  Port=2  VectorParamsAs1DForOutWhenUnconnected=off
  wires:
  abc2alphabeta/2(beta) -> ug_beta/1  "u_grid_beta"
  abc2alphabeta/1(alpha) -> ug_alpha/1  "u_grid_alpha"
  ug_a/1 -> abc2alphabeta/1(a)
  ug_b/1 -> abc2alphabeta/2(b)
  ug_c/1 -> abc2alphabeta/3(c)

== system frt_dqpll/AFE_control/afe_control/grid_voltage_phase_lock_loops/dq_pll/pll_stageA/sequences ==
  u_grid_alpha : Inport
  u_grid_beta : Inport  Port=2
  gamma_grid : Inport  Port=3
  alphabeta2xieta : Subsystem
  u_grid_pos_xi : Outport
  u_grid_pos_eta : Outport  Port=2
  wires:
  alphabeta2xieta/1(xi) -> u_grid_pos_xi/1  "u_grid_pos_xi"
  alphabeta2xieta/2(eta) -> u_grid_pos_eta/1  "u_grid_pos_eta"
  u_grid_alpha/1 -> alphabeta2xieta/1(alpha)  "u_grid_alpha"
  u_grid_beta/1 -> alphabeta2xieta/2(beta)  "u_grid_beta"
  gamma_grid/1 -> alphabeta2xieta/3(gamma)  "phase_grid"

== system frt_dqpll/AFE_control/afe_control/grid_voltage_phase_lock_loops/dq_pll/pll_stageB/double_integrator_observer ==
  theta : Inport
  Gain : Gain  Gain=Ldrso  Multiplication=Matrix(K*u)
  Gain1 : Gain  Gain=Adrso  Multiplication=Matrix(K*u)
  Gain2 : Gain  Gain=Crso  Multiplication=Matrix(K*u)
  Selector : Selector  InputPortWidth=2  IndexOptions=Index vector (dialog)  Indices=2  OutputSizes=1
  Sum : Sum  Inputs=-+|
  Sum1 : Sum  Inputs=|++
  Unit Delay : UnitDelay  SampleTime=-1  HasFrameUpgradeWarning=on
  bounder1 : MATLAB Function  TreatAsAtomicUnit=on
  bounder2 : MATLAB Function  TreatAsAtomicUnit=on
  omega_hat : Outport
  wires:
  Gain/1 -> Sum1/1
  Selector/1 -> omega_hat/1
  Gain2/1 -> bounder2/1(u)  "theta_hat"
  Gain1/1 -> Sum1/2
  Sum1/1 -> Unit Delay/1
  Sum/1 -> bounder1/1(u)  "e"
  Unit Delay/1 -> Gain1/1, Selector/1, Gain2/1
  bounder1/1(y) -> Gain/1  "e_bounded"
  bounder2/1(y) -> Sum/1  "theta_hat_bounded"
  theta/1 -> Sum/2

== system frt_dqpll/AFE_control/afe_control/grid_voltage_phase_lock_loops/dq_pll/pll_stageB/scheduled-p-gain ==
  In1 : Inport
  Switch : Switch  Criteria=u2 > Threshold  Threshold=0.5  SaturateOnIntegerOverflow=off  InputSameDT=off
  kp1 : Gain  Gain=pll_p  SaturateOnIntegerOverflow=on  OutDataTypeStr=Inherit: Same as input  ParamDataTypeStr=Inherit: Same as input
  kp3 : Gain  Gain=pll_p_frt  SaturateOnIntegerOverflow=on  OutDataTypeStr=Inherit: Same as input  ParamDataTypeStr=Inherit: Same as input
  Out2 : Outport
  wires:
  kp3/1 -> Switch/1
  kp1/1 -> Switch/3
  [frt_active_mod1] -> Switch/2
  In1/1 -> kp1/1, kp3/1
  Switch/1 -> Out2/1

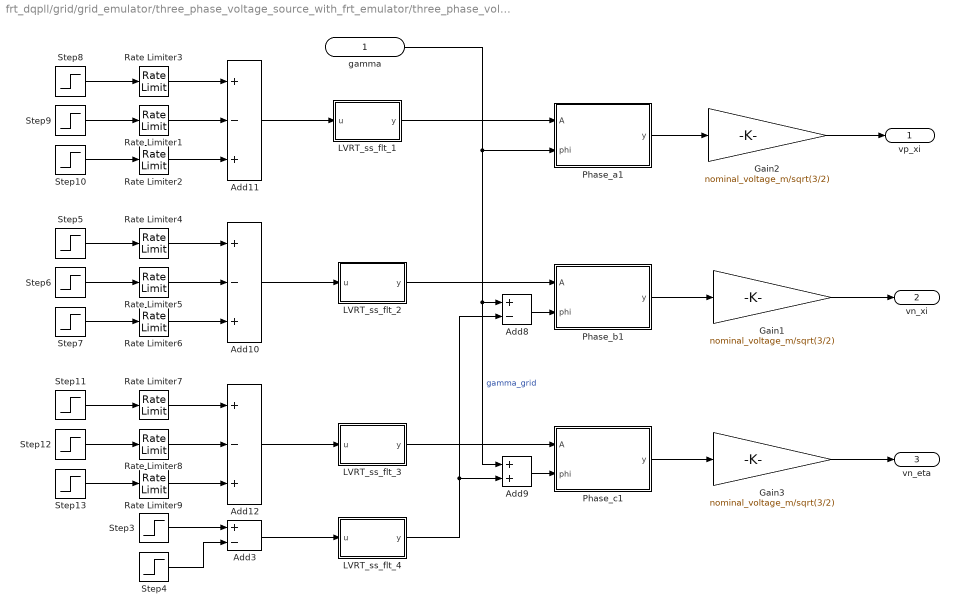
== system frt_dqpll/grid/grid_emulator/three_phase_voltage_source_with_frt_emulator/three_phase_voltage_source_emulator/voltage_reference1/voltage_dource_with_frt ==
  gamma : Inport
  Add10 : Sum  Inputs=+-+
  Add11 : Sum  Inputs=+-+
  Add12 : Sum  Inputs=+-+
  Add3 : Sum  Inputs=+-
  Add8 : Sum  Inputs=+-
  Add9 : Sum
  Gain1 : Gain  Gain=nominal_voltage_m/sqrt(3/2)
  Gain2 : Gain  Gain=nominal_voltage_m/sqrt(3/2)
  Gain3 : Gain  Gain=nominal_voltage_m/sqrt(3/2)
  LVRT_ss_flt_1 : Subsystem
  LVRT_ss_flt_2 : Subsystem
  LVRT_ss_flt_3 : Subsystem
  LVRT_ss_flt_4 : Subsystem
  Phase_a1 : MATLAB Function  TreatAsAtomicUnit=on
  Phase_b1 : MATLAB Function  TreatAsAtomicUnit=on
  Phase_c1 : MATLAB Function  TreatAsAtomicUnit=on
  Rate Limiter{1..9} (9 alike) : RateLimiter  RisingSlewLimit=Vemu_ref_norm_m/t_ramp_m  FallingSlewLimit=-Vemu_ref_norm_m/t_ramp_m  SampleTimeMode=inherited
  Step10 : Step  Time=end_time_LVRT_m  After=Vemu_ref_norm_m*(1-Amplitude_U_m)  SampleTime=0
  Step11 : Step  Time=0  After=Vemu_ref_norm_m  SampleTime=0
  Step12 : Step  Time=start_time_LVRT_m  After=Vemu_ref_norm_m*(1-Amplitude_W_m)  SampleTime=0
  Step13 : Step  Time=end_time_LVRT_m  After=Vemu_ref_norm_m*(1-Amplitude_W_m)  SampleTime=0
  Step3 : Step  Time=start_time_LVRT  After=Phase_shift_m  SampleTime=0
  Step4 : Step  Time=end_time_LVRT_m  After=Phase_shift_m  SampleTime=0
  Step5 : Step  Time=0  After=Vemu_ref_norm_m  SampleTime=0
  Step6 : Step  Time=start_time_LVRT_m  After=Vemu_ref_norm_m*(1-Amplitude_V_m)  SampleTime=0
  Step7 : Step  Time=end_time_LVRT_m  After=Vemu_ref_norm_m*(1-Amplitude_V_m)  SampleTime=0
  Step8 : Step  Time=0  After=Vemu_ref_norm_m  SampleTime=0
  Step9 : Step  Time=start_time_LVRT_m  After=Vemu_ref_norm_m*(1-Amplitude_U_m)  SampleTime=0
  vp_xi : Outport  VectorParamsAs1DForOutWhenUnconnected=off
  vn_xi : Outport  Port=2  VectorParamsAs1DForOutWhenUnconnected=off
  vn_eta : Outport  Port=3  VectorParamsAs1DForOutWhenUnconnected=off
  wires:
  Gain3/1 -> vn_eta/1
  Gain1/1 -> vn_xi/1
  Gain2/1 -> vp_xi/1
  Add3/1 -> LVRT_ss_flt_4/1(u)
  Step4/1 -> Add3/2
  Step3/1 -> Add3/1
  Phase_c1/1(y) -> Gain3/1
  Phase_b1/1(y) -> Gain1/1
  Phase_a1/1(y) -> Gain2/1
  Rate Limiter7/1 -> Add12/1
  Step11/1 -> Rate Limiter7/1
  Rate Limiter9/1 -> Add12/3
  Step13/1 -> Rate Limiter9/1
  Rate Limiter8/1 -> Add12/2
  Step12/1 -> Rate Limiter8/1
  Rate Limiter6/1 -> Add10/3
  Rate Limiter5/1 -> Add10/2
  Rate Limiter4/1 -> Add10/1
  Rate Limiter2/1 -> Add11/3
  Rate Limiter1/1 -> Add11/2
  Rate Limiter3/1 -> Add11/1
  Add11/1 -> LVRT_ss_flt_1/1(u)
  Step10/1 -> Rate Limiter2/1
  Step9/1 -> Rate Limiter1/1
  Step8/1 -> Rate Limiter3/1
  Step7/1 -> Rate Limiter6/1
  Step6/1 -> Rate Limiter5/1
  Step5/1 -> Rate Limiter4/1
  Add10/1 -> LVRT_ss_flt_2/1(u)
  Add8/1 -> Phase_b1/2(phi)
  Add9/1 -> Phase_c1/2(phi)
  gamma/1 -> Phase_a1/2(phi), Add8/1, Add9/1  "gamma_grid"
  Add12/1 -> LVRT_ss_flt_3/1(u)
  LVRT_ss_flt_1/1(y) -> Phase_a1/1(A)
  LVRT_ss_flt_2/1(y) -> Phase_b1/1(A)
  LVRT_ss_flt_3/1(y) -> Phase_c1/1(A)
  LVRT_ss_flt_4/1(y) -> Add8/2, Add9/2
